simulink model "Trajectory_Tracking_Live"  (R2020a)
settings: Solver=VariableStepAuto  StartTime=0.0  StopTime=10.0  RelTol=1e-3
settings Model: Creator=Jeffrey  LastModifiedBy=Jeffrey

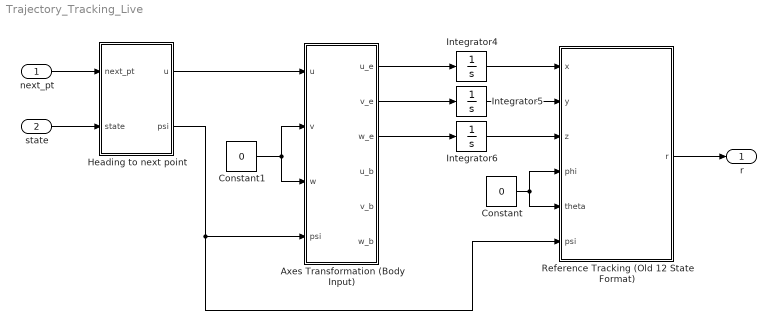
== system Trajectory_Tracking_Live ==
  next_pt : Inport
  state : Inport  Port=2
  Axes Transformation (Body Input) : MATLAB Function  TreatAsAtomicUnit=on
  Constant : Constant  Value=0
  Constant1 : Constant  Value=0
  Heading to next point : MATLAB Function  TreatAsAtomicUnit=on
  Integrator4 : Integrator
  Integrator5 : Integrator
  Integrator6 : Integrator  InitialCondition=1
  Reference Tracking (Old 12 State Format) : MATLAB Function  TreatAsAtomicUnit=on
  r : Outport
  wires:
  Reference Tracking (Old 12 State Format)/1(r) -> r/1
  Axes Transformation (Body Input)/1(u_e) -> Integrator4/1
  Axes Transformation (Body Input)/3(w_e) -> Integrator6/1
  Axes Transformation (Body Input)/2(v_e) -> Integrator5/1
  next_pt/1 -> Heading to next point/1(next_pt)
  state/1 -> Heading to next point/2(state)
  Heading to next point/2(psi) -> Axes Transformation (Body Input)/4(psi), Reference Tracking (Old 12 State Format)/6(psi)
  Integrator4/1 -> Reference Tracking (Old 12 State Format)/1(x)
  Integrator5/1 -> Reference Tracking (Old 12 State Format)/2(y)
  Integrator6/1 -> Reference Tracking (Old 12 State Format)/3(z)
  Constant/1 -> Reference Tracking (Old 12 State Format)/4(phi), Reference Tracking (Old 12 State Format)/5(theta)
  Heading to next point/1(u) -> Axes Transformation (Body Input)/1(u)
  Constant1/1 -> Axes Transformation (Body Input)/2(v), Axes Transformation (Body Input)/3(w)

== matlab function Trajectory_Tracking_Live/Heading to next point ==
  data: next_pt input; u output; state input; psi output
%% Always point to next point
function [u,psi] = fcn(next_pt,state)
x_curr = state(1);
y_curr = state(2);
x_next = next_pt(1);
y_next = next_pt(2);

persistent psi
psi = 0;

%Get heading angle (+ve is counter-clockwise)
psi_next = atan2( (x_next-x_curr),(y_next-y_curr) );

% To stop sudden 360 rotations assuming smooth trajectories NEEDS FIXING
if psi_next - psi> pi %jumps from -ve to +ve 

    psi_next = -pi - (pi-psi_next);

elseif psi_next - psi < -pi %jumps from +ve to -ve

    psi_next = pi + (pi+psi_next);

end

psi = psi_next;
u   = 0.5;

end

== matlab function Trajectory_Tracking_Live/Axes Transformation (Body Input) ==
  data: u input; u_e output; v input; w input; v_e output; w_e output; psi input; u_b output; v_b output; w_b output
function [u_e,v_e,w_e,u_b,v_b,w_b] = fcn(u, v, w, psi)

%rotating uvw vector (assume input u v w in body frame)
a=0; b=0; c=psi;
T_roll = [ 1, 0      , 0    ;
         0, cos(a) , sin(a) ;
         0, -sin(a), cos(a) ];
     
T_pitch = [cos(b),0,-sin(b) ;
        0     ,1,0       ;
        sin(b),0,cos(b)  ];
    
T_yaw = [cos(c) ,sin(c),0;
        -sin(c),cos(c),0;
        0      ,0     ,1];

T_BE = T_roll * T_pitch * T_yaw;

V_e = T_BE^-1 * [u;v;w];

u_e = V_e(1);
v_e = V_e(2);
w_e = V_e(3);

u_b = u;
v_b = v;
w_b = w;

== matlab function Trajectory_Tracking_Live/Reference Tracking (Old 12 State Format) ==
  data: x input; y input; z input; r output; phi input; theta input; psi input
function r = fcn(x,y,z,phi,theta,psi)

r = zeros(12,1);
% reference output
r(1) = x;
r(2) = y;
r(3) = z;
r(7) = phi;
r(8) = theta;
r(9) = psi;
